simulink model "GearBox"  (Simulink 8.3)
settings: Solver=ode45  StartTime=0.0  StopTime=10.0  RelTol=1e-3
undefined symbols (not defined in the file): i
settings Model: Creator=Administrator  LastModifiedBy=Administrator
settings DataIOCC: SignalLoggingSaveFormat=Dataset
settings DebuggingCC: UnderspecifiedInitializationDetection=Simplified  StateNameClashWarn=none
settings GRTTargetCC: CombineOutputUpdateFcns=on  GRTInterface=off

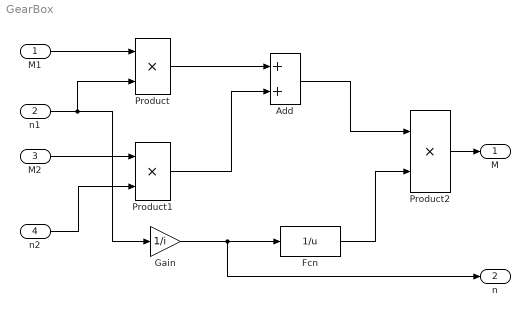
== system GearBox ==
  M1 : Inport
  n1 : Inport  Port=2
  M2 : Inport  Port=3
  n2 : Inport  Port=4
  Add : Sum
  Fcn : Fcn  Expr=1/u
  Gain : Gain  Gain=1/i
  Product : Product
  Product1 : Product
  Product2 : Product
  M : Outport
  n : Outport  Port=2
  wires:
  M1/1 -> Product/1
  n1/1 -> Gain/1, Product/2
  Product/1 -> Add/1
  M2/1 -> Product1/1
  n2/1 -> Product1/2
  Product1/1 -> Add/2
  Gain/1 -> n/1, Fcn/1
  Add/1 -> Product2/1
  Fcn/1 -> Product2/2
  Product2/1 -> M/1
